simulink model "RectifierBuck"  (R2018a)
settings: Solver=VariableStepAuto  StartTime=0.0  StopTime=10  RelTol=1e-3
libraries: powerlib x15, powerlib_meascontrol x1
settings Model: Creator=user  LastModifiedBy=user

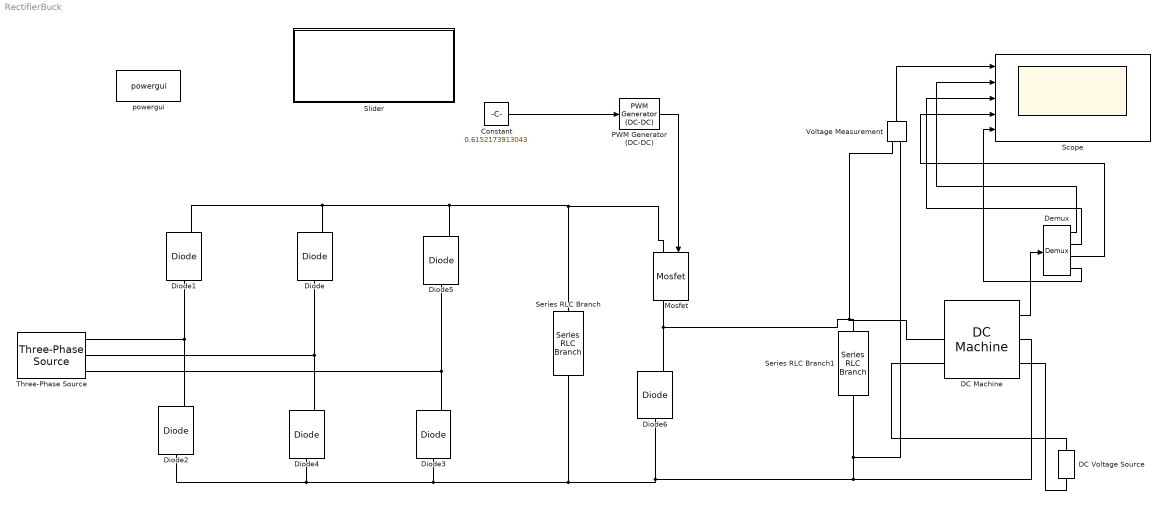
== system RectifierBuck ==
  Constant : Constant  Value=0.6152173913043
  DC Machine : powerlib/Machines/DC Machine  PresetModel=No  MechanicalLoad=Torque TL  FieldType=Wound  ShowDetailedParameters=on  MeasurementBus=on  RLa="[ 0.8  0.0125]"  RLf="[ 210  23]"  Laf=1.8  MachineConstant=Torque constant (N.m/A)  Ke=1.8  Kt=1.8  J=1  Bm=0  Tf=0  w0=0  Ifinit=0  TsPowergui=0  TsBlock=-1
  DC Voltage Source : powerlib/Electrical Sources/DC Voltage Source  Amplitude=100  Measurements=None
  Demux : Demux
  Diode{,1..6} (7 alike) : powerlib/Power Electronics/Diode  Ron=0.001  Lon=0  Vf=0.8  IC=0  UseSnubber=0  Rs=500  Cs=250e-9  Measurements=on
  Mosfet : powerlib/Power Electronics/Mosfet  Ron=0.1  Lon=0  Rd=0.01  Vfd=0  IC=0  Rs=1e5  Cs=inf  Measurements=on
  PWM Generator (DC-DC) : powerlib_meascontrol/Pulse & Signal Generators/PWM Generator (DC-DC)  Fsw=500  Ts=0
  Scope : Scope  NumInputPorts=5
  Series RLC Branch : powerlib/Elements/Series RLC Branch  LConnTagsString=__new0  RConnTagsString=__new0  BranchType=C  Resistance=1  Inductance=1e-3  SetiL0=off  InitialCurrent=0  Capacitance=0.001  Setx0=off  InitialVoltage=0  Measurements=None
  Series RLC Branch1 : powerlib/Elements/Series RLC Branch  LConnTagsString=__new0  RConnTagsString=__new0  BranchType=C  Resistance=1  Inductance=1e-3  SetiL0=off  InitialCurrent=0  Capacitance=0.0001  Setx0=off  InitialVoltage=0  Measurements=None
  Slider : Subsystem  DialogController=hmiCreateDDGDialog  IsWebBlock=on  mask(MWDashboardBlock){webBlockId=4ef0fdb7-b675-434c-9747-e633bbe24ef6, webBlockType=slider, ShowInLibBrowser=on, ShowInitialText=on, HMISrcModelName=RectifierBuck}
      mask prompts: webBlockId "WebBlock Id"; webBlockType "WebBlock Type"; HMISrcModelName "Source Model"
      mask help: SimulinkHMI:dialogs:SliderDialogDesc
      mask Help: helpview([docroot '/mapfiles/simulink.map'], 'hmi_slider')
      mask Display:
      | if strcmp(get_param(bdroot(gcb),'BlockDiagramType'), 'library')
      |     image([(matlabroot) '/toolbox/simulink/hmi/icons/Slider.png']);
      | end
  Three-Phase Source : powerlib/Electrical Sources/Three-Phase Source  InternalConnection=Yg  VoltagePhases=off  Voltage=140  PhaseAngle=0  Voltage_phases=[25e3 25e3 25e3]/sqrt(3)  PhaseAngles_phases=[0 -120 +120]  Frequency=50  NonIdealSource=on  SpecifyImpedance=off  Resistance=0  Inductance=0  ShortCircuitLevel=100e6  BaseVoltage=0  XRratio=7  BusType=swing  Pref=10e3  Qref=0  Prefabc=[10e3, 10e3, 10e3]  Qrefabc=[0, 0, 0]  Qmin=-inf  Qmax=inf
  Voltage Measurement : powerlib/Measurements/Voltage Measurement  PhasorSimulation=off  OutputType=Complex  PSBequivalent=0
  powergui : powerlib/powergui  Priority=1  SimulationMode=Continuous  SampleTime=50e-6  frequency=60  Iterations=50  frequencyindice=0  Pbase=100e6  ErrMax=1e-4  UnitsV=kV  UnitsW=MW  buscounter=0  FunctionMessages=off  echomessages=off  EnableUseOfTLC=off  CurrentSourceSwitches=off  DisableSnubberDevices=off  DisableRonSwitches=off  DisableVfSwitches=off  DisplayEquations=off  SolverType=Tustin/Backward Euler (TBE)  Interpol=off  ExternalGateDelay=off  methode=off  Ts=100  x0status=blocks  SPID=on  SwTol=0  HookPort=off  RestoreLinks=warning  ResistiveCurrentMeasurement=off  Frange=[0:2:500]  Ylog=off  Xlog=on  ShowGrid=off  save=off  variable=ZData  structure=0  ZoomFFT=off  StartTime=0.0  cycles=1  DisplayStyle=1  fundamental=60  FreqAxis=off  MaxFrequency=1000  frequencyindicesteady=1  RmsSteady=1  display=off
  wires:
  PWM Generator (DC-DC)/1 -> Mosfet/1
  Constant/1 -> PWM Generator (DC-DC)/1
  Voltage Measurement/1 -> Scope/1
  Demux/1 -> Scope/2
  DC Machine/1 -> Demux/1
  Demux/2 -> Scope/3
  Demux/3 -> Scope/4
  Demux/4 -> Scope/5
  connections:
  Diode1/LConn1 -- Three-Phase Source/RConn1 -- Diode2/RConn1
  Diode/LConn1 -- Three-Phase Source/RConn2 -- Diode4/RConn1
  Diode5/LConn1 -- Three-Phase Source/RConn3 -- Diode3/RConn1
  Diode1/RConn1 -- Mosfet/LConn1 -- Series RLC Branch/LConn1 -- Diode5/RConn1 -- Diode/RConn1
  Diode2/LConn1 -- Diode3/LConn1 -- Voltage Measurement/LConn2 -- Series RLC Branch1/RConn1 -- DC Machine/RConn1 -- Diode6/LConn1 -- Series RLC Branch/RConn1 -- Diode4/LConn1
  Voltage Measurement/LConn1 -- Mosfet/RConn1 -- Diode6/RConn1 -- Series RLC Branch1/LConn1 -- DC Machine/LConn1
  DC Voltage Source/RConn1 -- DC Machine/LConn2
  DC Voltage Source/LConn1 -- DC Machine/RConn2

== system RectifierBuck/Slider ==
